simulink model "Q9"  (R2020b)
settings: Solver=VariableStepAuto  StartTime=0.0  StopTime=0.1  RelTol=1e-3
libraries: powerlib x3
settings Model: Creator=Huzai  LastModifiedBy=Huzai

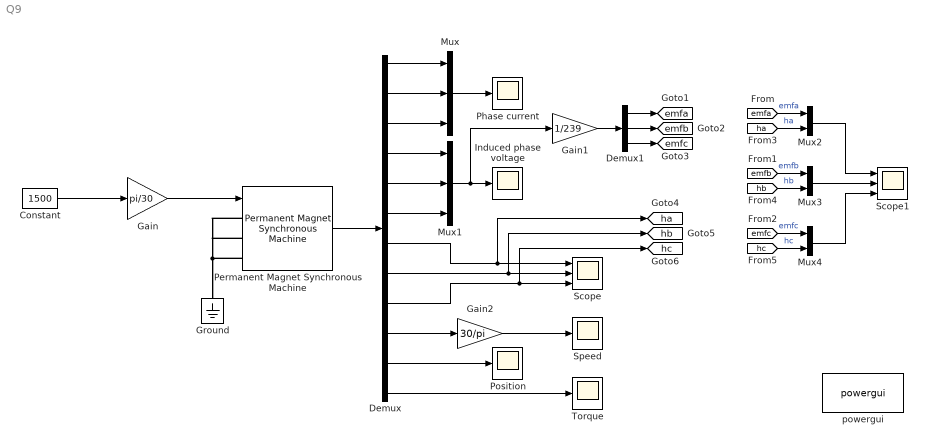
== system Q9 ==
  Constant : Constant  Value=1500
  Demux : Demux  Outputs=12
  Demux1 : Demux  Outputs=3
  Gain : Gain  Gain=pi/30
  Gain1 : Gain  Gain=1/239
  Gain2 : Gain  Gain=30/pi
  Ground : powerlib/Elements/Ground  LConnTagsString=a
  Induced phase voltage : Scope
  Mux : Mux  Inputs=3
  Mux1 : Mux  Inputs=3
  Mux2 : Mux  Inputs=2
  Mux3 : Mux  Inputs=2
  Mux4 : Mux  Inputs=2
  Permanent Magnet Synchronous Machine : powerlib/Machines/Permanent Magnet Synchronous Machine  NbPhases=3  FluxDistribution=Trapezoidal  RotorType=Round  MechanicalLoad=Speed w  PresetModel=No  ShowDetailedParameters=on  MeasurementBus=off  Resistance=8  Inductance=5.68e-3  dqInductances=[8.5e-3,8.5e-3]  La=0.000395  MachineConstant=Flux linkage established by magnets (V.s)  Flux=0.37973  VoltageCst=318.1219  TorqueCst=3.0378  Flat=120  Mechanical=[0.0027 0.0004924 4 0]  PolePairs=4  InitialConditions=[0,0, 0,0]  InitialConditions5ph=[0 0 0 0 0 0]  RefAngle=90 degrees behind phase A axis (modified Park)  IterativeDiscreteModel=Trapezoidal non iterative  TsBlock=-1  TsPowergui=0
  Phase current : Scope
  Position : Scope
  Scope : Scope  NumInputPorts=3
  Scope1 : Scope  NumInputPorts=3
  Speed : Scope
  Torque : Scope
  powergui : powerlib/powergui  Priority=1  SimulationMode=Continuous  SampleTime=50e-6  frequency=60  Iterations=50  frequencyindice=0  Pbase=100e6  ErrMax=1e-4  UnitsV=kV  UnitsW=MW  buscounter=0  FunctionMessages=off  echomessages=off  EnableUseOfTLC=off  CurrentSourceSwitches=off  DisableSnubberDevices=off  DisableRonSwitches=off  DisableVfSwitches=off  DisplayEquations=off  AutomaticDiscreteSolvers=off  SolverType=Tustin/Backward Euler (TBE)  Interpol=off  ExternalGateDelay=off  methode=off  Ts=100  x0status=blocks  SPID=on  SwTol=0  HookPort=off  NonlinearTolerance=1e-4  nMaxIteration=100  ContinueOnMaxIteration=off  RestoreLinks=warning  ResistiveCurrentMeasurement=off  Frange=[0:2:500]  Ylog=off  Xlog=on  ShowGrid=off  save=off  variable=ZData  structure=0  ZoomFFT=off  StartTime=0.0  cycles=1  DisplayStyle=1  fundamental=60  FreqAxis=off  MaxFrequency=1000  frequencyindicesteady=1  RmsSteady=1  display=off
  tag scope: emfa=global, emfb=global, emfc=global, ha=global, hb=global, hc=global
  wires:
  Gain/1 -> Permanent Magnet Synchronous Machine/1
  Constant/1 -> Gain/1
  Permanent Magnet Synchronous Machine/1 -> Demux/1
  Demux/1 -> Mux/1
  Demux/2 -> Mux/2
  Demux/3 -> Mux/3
  Demux/4 -> Mux1/1
  Demux/5 -> Mux1/2
  Demux/6 -> Mux1/3
  Mux/1 -> Phase current/1
  Mux1/1 -> Gain1/1, Induced phase voltage/1
  Gain1/1 -> Demux1/1
  Demux1/1 -> [emfa]
  Demux1/2 -> [emfb]
  Demux1/3 -> [emfc]
  Demux/8 -> [hb], Scope/2
  Demux/7 -> Scope/1, [ha]
  Demux/9 -> [hc], Scope/3
  Demux/10 -> Gain2/1
  Gain2/1 -> Speed/1
  Demux/11 -> Position/1
  Demux/12 -> Torque/1
  [emfa] -> Mux2/1  "emfa"
  [ha] -> Mux2/2  "ha"
  [emfb] -> Mux3/1  "emfb"
  [hb] -> Mux3/2  "hb"
  [emfc] -> Mux4/1  "emfc"
  [hc] -> Mux4/2  "hc"
  Mux2/1 -> Scope1/1
  Mux3/1 -> Scope1/2
  Mux4/1 -> Scope1/3
  connections:
  Permanent Magnet Synchronous Machine/LConn3 -- Permanent Magnet Synchronous Machine/LConn1 -- Permanent Magnet Synchronous Machine/LConn2 -- Ground/LConn1
